simulink model "ReadFromServo_test"  (R2014b)
settings: Solver=ode3  StartTime=0.0  StopTime=30  RelTol=1e-3
libraries: BeagleBoneBlackCom x1
settings Model: SimulationMode=external  Creator=Sebastian  LastModifiedBy=Sebastian
settings OptimizationCC: OptimizeModelRefInitCode=on  LifeSpan=1  MaxStackSize=64
settings HardwareCC: ProdLargestAtomicInteger=Long  ProdLargestAtomicFloat=Double  ProdEndianess=LittleEndian  ProdHWDeviceType=ARM Compatible->ARM Cortex
settings RTWCC: SystemTargetFile=ert.tlc  TLCOptions=-aInlineSetEventsForThisBaseRateFcn=TLC_FALSE -aSuppressMultiTaskScheduler=TLC_FALSE  TemplateMakefile=ert_default_tmf  Description=Embedded Coder  GenerateReport=on  ProcessScript=ert_make_rtw_hook  Toolchain=Linaro Toolchain v4.8  BuildConfiguration=Specify  IncludeHyperlinkInReport=on  LaunchReport=on  GenerateTraceReport=on  GenerateTraceReportSl=on  GenerateTraceReportSf=on  GenerateTraceReportEml=on  GenerateCodeMetricsReport=on
settings CodeAppCC: IgnoreCustomStorageClasses=off

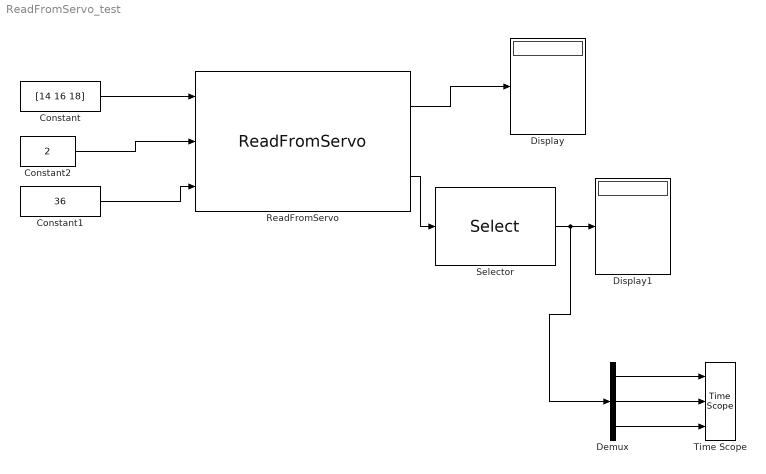
== system ReadFromServo_test ==
  Constant : Constant  Value=[14 16 18]  OutDataTypeStr=uint8  SampleTime=-1
  Constant1 : Constant  Value=36  OutDataTypeStr=uint8  SampleTime=-1
  Constant2 : Constant  Value=2  OutDataTypeStr=uint8  SampleTime=-1
  Demux : Demux  Outputs=3
  Display : Display
  Display1 : Display
  ReadFromServo : BeagleBoneBlackCom/ReadFromServo
  Selector : Selector  IndexMode=Zero-based  InputPortWidth=18  IndexOptions=Starting index (dialog)  Indices=0  OutputSizes=3
  Time Scope : TimeScope  DefaultConfigurationName=spbscopes.TimeScopeBlockCfg  NumInputPorts=3
  wires:
  Constant2/1 -> ReadFromServo/2
  ReadFromServo/1 -> Display/1
  Constant/1 -> ReadFromServo/1
  Constant1/1 -> ReadFromServo/3
  ReadFromServo/2 -> Selector/1
  Selector/1 -> Demux/1, Display1/1
  Demux/1 -> Time Scope/1
  Demux/2 -> Time Scope/2
  Demux/3 -> Time Scope/3
